simulink model "LogModel"  (R2014a)
settings: Solver=ode3  StartTime=0.0  StopTime=Inf  RelTol=1e-3
StartFcn:
  | localAddEventListener
libraries: iWalkerLib x2
settings Model: Creator=Brian  LastModifiedBy=Brian
settings OptimizationCC: BlockReduction=off

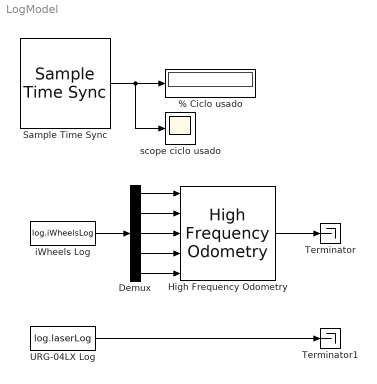
== system LogModel ==
  % Ciclo usado : Display
      settings: Decimation=100
  Demux : Demux  Outputs=5
  High Frequency Odometry : iWalkerLib/High Frequency Odometry
  Sample Time Sync : iWalkerLib/Sample Time Sync  Priority=1  SampleTime=0.01
  Terminator : Terminator
  Terminator1 : Terminator
  URG-04LX Log : FromWorkspace  Priority=3  VariableName=log.laserLog  SampleTime=0.5  Interpolate=off  OutputAfterFinalValue=Setting to zero
  iWheels Log : FromWorkspace  Priority=2  VariableName=log.iWheelsLog  SampleTime=0.01  Interpolate=off  OutputAfterFinalValue=Setting to zero
  scope ciclo usado : Scope
      settings: TimeRange=0.7489177489177488  YMin=0  YMax=250
  wires:
  Sample Time Sync/1 -> scope ciclo usado/1, % Ciclo usado/1
  URG-04LX Log/1 -> Terminator1/1
  Demux/1 -> High Frequency Odometry/1
  High Frequency Odometry/1 -> Terminator/1
  iWheels Log/1 -> Demux/1
  Demux/2 -> High Frequency Odometry/2
  Demux/3 -> High Frequency Odometry/3
  Demux/4 -> High Frequency Odometry/4
  Demux/5 -> High Frequency Odometry/5
